simulink model "sl_vessel"  (R2022a)
settings: Solver=VariableStepAuto  StartTime=0.0  StopTime=50  RelTol=1e-3
values from neighbouring files (symbols this model uses):
  accel = inf    [vessel.m]
  B = atand((L3/2)/L4)    [vessel.m]
  bf = double(svar.bf)    [vessel.m]
  bt = double(svar.bt)    [vessel.m]
  bvx = double(svar.bvx)    [vessel.m]
  bvy = double(svar.bvy)    [vessel.m]
  bw = double(svar.bw)    [vessel.m]
  I = 25    [vessel.m]
  L5 = sqrt(L4^2+(L3/2)^2)    [vessel.m]
  L6 = 0.4    [vessel.m]
  m = 60    [vessel.m]
  wlim = 5000    [vessel.m]
  wtlim = 6000    [vessel.m]
settings Model: Creator=mnks9  LastModifiedBy=mnks9

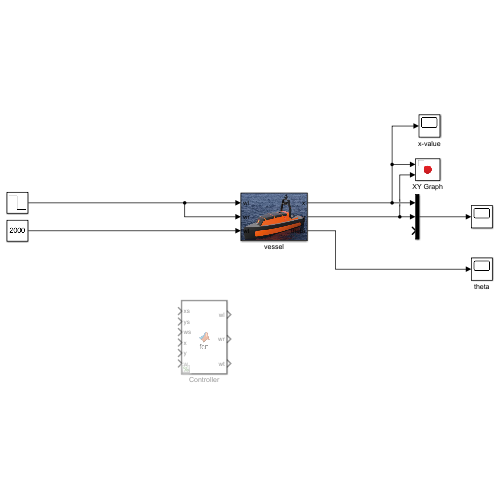
[thumbnail: Simulink's stored preview of the top-level diagram]
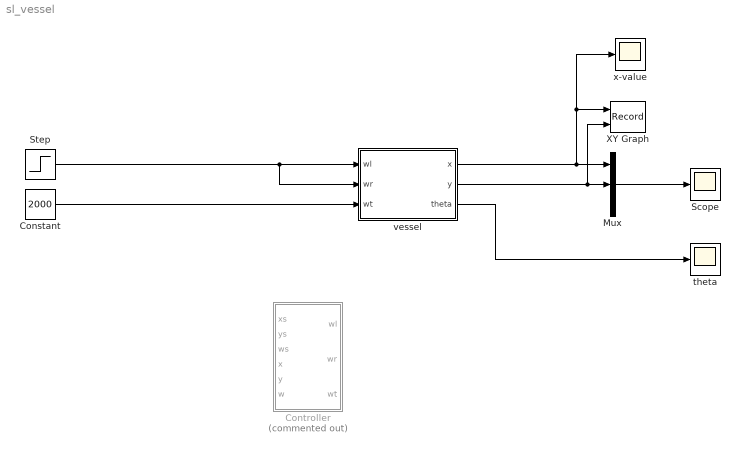
== system sl_vessel ==
  Constant : Constant  Value=2000
  Controller : MATLAB Function  Commented=on  TreatAsAtomicUnit=on
  Mux : Mux  Inputs=3
  Scope : Scope
  Step : Step  Time=25  Before=4000  After=0  SampleTime=0
  XY Graph : Record  FileSettingsInternal="{\"entries\":[{\"content\":{\"excelSettings\":{\"content\":{},\"type\":\"Streamout.ExcelSettings\"}},\"type\":\"Streamout.FileSettingStorage\",\"uuid\":\"077adc5f-c83b-407b-861b-79d7fc127e89\"}],\"packageUris\":[\"http://schema.mathworks.com/mf0/streamout_blocks/R2020a\"],\"version\":\"1.0\"}"  Layout=[1 1]  SignalsInternal="{\"entries\":[{\"content\":{\"signals\":[{\"content\":{\"blockPath\":[\"sl_vessel/XY Graph\"],\"channel\":[],\"dimensions\":[1],\"domain\":\"sl_vessel/XY Graph\",\"lineColor\":\"#a2142f\",\"plots\":[1],\"port\":1,\"sid\":[\"\"],\"signalID\":42,\"signalName\":\"vessel:1\"},\"type\":\"RecordBlkView.Signal\",\"uuid\":\"51d972bf-d378-48b9-8560-0daaad8fc76a\"},{\"content\":{\"blockPath\":[\"sl_vessel/XY Graph\"],\"channel\":[],\"dimensions\":[1],\"domain\":\"sl_vessel/XY Graph\",\"lineColor\":\"#139fff\",\"plots\":[1],\"port\":2,\"sid\":[\"\"],\"signalID\":46,\"signalName\":\"vessel:2\"},\"type\":\"RecordBlkView.Signal\",\"uuid\":\"d4cbe20f-f084-4d84-af59-733677b681e9\"}]},\"type\":\"RecordBlkView.InputSignals\",\"uuid\":\"f14646e1-6c27-4682-8f64-9d52d7544a54\"}],\"packageUris\":[\"http://schema.mathworks.com/mf0/streamout_blocks/R2020a\"],\"version\":\"1.0\"}"  VisualizationBindings="{\"xyplotplugin\":{\"info\":[{\"series\":[{\"bindingParametersList\":[{\"parameter\":\"X-Axis\",\"signalID\":42,\"signalName\":\"vessel:1\"},{\"parameter\":\"Y-Axis\",\"signalID\":46,\"signalName\":\"vessel:2\"}],\"seriesID\":10976}],\"subplotID\":1}]}}"  CompatibilityTag=XY
  theta : Scope
  vessel : Subsystem
      mask Display: image('C:\Users\mnks9\OneDrive\ELE306\Matlab\library\vessel.jpg'); % Use "Edit Image" on toolstrip to change.
  x-value : Scope
  wires:
  Mux/1 -> Scope/1
  vessel/3(theta) -> theta/1
  Constant/1 -> vessel/3(wt)
  Step/1 -> vessel/2(wr), vessel/1(wl)
  vessel/1(x) -> x-value/1, XY Graph/1, Mux/1
  vessel/2(y) -> XY Graph/2, Mux/2

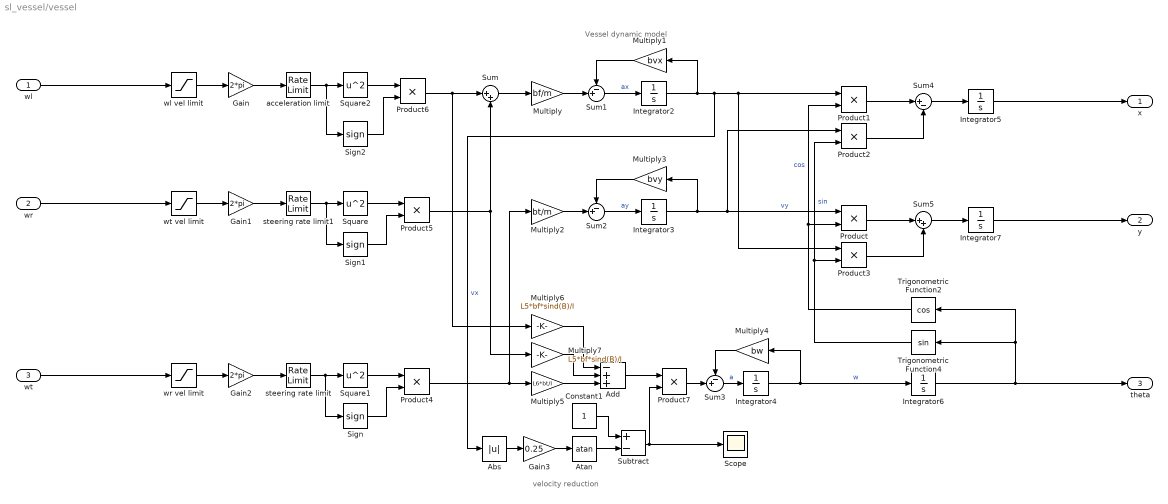
== system sl_vessel/vessel ==
  note: Vessel dynamic model
  note: velocity reduction
  wl : Inport
  wr : Inport  Port=2
  wt : Inport  Port=3
  Abs : Abs  SaturateOnIntegerOverflow=off
  Add : Sum  Inputs=-++
  Atan : Trigonometry  Operator=atan
  Constant1 : Constant
  Gain : Gain  Gain=2*pi
  Gain1 : Gain  Gain=2*pi
  Gain2 : Gain  Gain=2*pi
  Gain3 : Gain  Gain=0.25
  Integrator{2..7} (6 alike) : Integrator
  Multiply : Gain  Gain=bf/m
  Multiply1 : Gain  Gain=bvx
  Multiply2 : Gain  Gain=bt/m
  Multiply3 : Gain  Gain=bvy
  Multiply4 : Gain  Gain=bw
  Multiply5 : Gain  Gain=L6*bt/I
  Multiply6 : Gain  Gain=L5*bf*sind(B)/I
  Multiply7 : Gain  Gain=L5*bf*sind(B)/I
  Product{,1..6} (7 alike) : Product  RndMeth=Zero
  Product7 : Product
  Scope : Scope
  Sign : Signum
  Sign1 : Signum
  Sign2 : Signum
  Square : Math  Operator=square
  Square1 : Math  Operator=square
  Square2 : Math  Operator=square
  Subtract : Sum  Inputs=+-
  Sum : Sum  Inputs=|++
  Sum1 : Sum  Inputs=-+|
  Sum2 : Sum  Inputs=-+|
  Sum3 : Sum  Inputs=-+|
  Sum4 : Sum  Inputs=|+-
  Sum5 : Sum  Inputs=|++
  Trigonometric Function2 : Trigonometry  Operator=cos
  Trigonometric Function4 : Trigonometry
  acceleration limit : RateLimiter  RisingSlewLimit=accel  FallingSlewLimit=-accel  SampleTimeMode=inherited
  steering rate limit : RateLimiter  RisingSlewLimit=accel  FallingSlewLimit=-accel  SampleTimeMode=inherited
  steering rate limit1 : RateLimiter  RisingSlewLimit=accel  FallingSlewLimit=-accel  SampleTimeMode=inherited
  wl vel limit : Saturate  UpperLimit=wlim  LowerLimit=-wlim
  wr vel limit : Saturate  UpperLimit=wtlim  LowerLimit=-wtlim
  wt vel limit : Saturate  UpperLimit=wlim  LowerLimit=-wlim
  x : Outport
  y : Outport  Port=2
  theta : Outport  Port=3
  wires:
  Integrator2/1 -> Abs/1, Product3/1, Product1/1, Multiply1/1  "vx"
  Product4/1 -> Multiply2/1, Multiply5/1
  Product1/1 -> Sum4/1
  Square/1 -> Product5/1
  Multiply2/1 -> Sum2/2
  Product6/1 -> Sum/1, Multiply6/1
  Product/1 -> Sum5/1
  acceleration limit/1 -> Sign2/1, Square2/1
  Square2/1 -> Product6/1
  Multiply5/1 -> Add/3
  Trigonometric Function2/1 -> Product/2, Product1/2  "cos"
  Product2/1 -> Sum4/2
  Product5/1 -> Multiply7/1, Sum/2
  wt/1 -> wr vel limit/1
  Sum2/1 -> Integrator3/1  "ay"
  Integrator6/1 -> Trigonometric Function2/1, Trigonometric Function4/1, theta/1
  steering rate limit/1 -> Sign/1, Square1/1
  Integrator3/1 -> Product2/1, Product/1, Multiply3/1  "vy"
  Integrator5/1 -> x/1
  wt vel limit/1 -> Gain1/1
  Sum3/1 -> Integrator4/1  "a"
  steering rate limit1/1 -> Sign1/1, Square/1
  Sum/1 -> Multiply/1
  wr vel limit/1 -> Gain2/1
  Trigonometric Function4/1 -> Product3/2, Product2/2  "sin"
  Sum5/1 -> Integrator7/1
  Gain/1 -> acceleration limit/1
  Sign2/1 -> Product6/2
  Multiply4/1 -> Sum3/1
  Constant1/1 -> Subtract/1
  Multiply6/1 -> Add/1
  Multiply1/1 -> Sum1/1
  wl/1 -> wl vel limit/1
  Sum4/1 -> Integrator5/1
  Sum1/1 -> Integrator2/1  "ax"
  Integrator4/1 -> Integrator6/1, Multiply4/1  "w"
  Square1/1 -> Product4/1
  Multiply3/1 -> Sum2/1
  Multiply7/1 -> Add/2
  Sign1/1 -> Product5/2
  Multiply/1 -> Sum1/2
  Gain1/1 -> steering rate limit1/1
  Integrator7/1 -> y/1
  Sign/1 -> Product4/2
  wl vel limit/1 -> Gain/1
  Abs/1 -> Gain3/1
  Subtract/1 -> Scope/1, Product7/2
  Add/1 -> Product7/1
  Gain3/1 -> Atan/1
  Gain2/1 -> steering rate limit/1
  Product3/1 -> Sum5/2
  Product7/1 -> Sum3/2
  Atan/1 -> Subtract/2
  wr/1 -> wt vel limit/1

== matlab function sl_vessel/Controller ==
  data: xs input; ys input; ws input; x input; wl output; y input; w input; wr output; wt output
function [wl, wr, wt]= fcn(xs,ys,ws,x,y,w)

wl = x;
